simulink library "slib_spectrum_analyser"  (R2020a)
settings: Solver=VariableStepAuto  StartTime=0.0  StopTime=10.0  RelTol=1e-3
libraries: hdlsllib x104, simulink x55, dsphdlxfrm x11, $bdroot x5
(part 3 of 3)

== system slib_spectrum_analyser/SSR Subset Converter/SSR Serializer Imag/Vector to SSR ==
  Vector : Inport
  Bit Concat : hdlsllib/Logic and Bit Operations/Bit Concat  numInputs=8
  Selector0 : Selector  InputPortWidth=8  IndexOptions=Index vector (dialog)  Indices=8  OutputSizes=1
  Selector1 : Selector  InputPortWidth=8  IndexOptions=Index vector (dialog)  Indices=7  OutputSizes=1
  Selector2 : Selector  InputPortWidth=8  IndexOptions=Index vector (dialog)  Indices=6  OutputSizes=1
  Selector3 : Selector  InputPortWidth=8  IndexOptions=Index vector (dialog)  Indices=5  OutputSizes=1
  Selector4 : Selector  InputPortWidth=8  IndexOptions=Index vector (dialog)  Indices=4  OutputSizes=1
  Selector5 : Selector  InputPortWidth=8  IndexOptions=Index vector (dialog)  Indices=3  OutputSizes=1
  Selector6 : Selector  InputPortWidth=8  IndexOptions=Index vector (dialog)  Indices=2  OutputSizes=1
  Selector7 : Selector  InputPortWidth=8  IndexOptions=Index vector (dialog)  Indices=1  OutputSizes=1
  SSR : Outport
  wires:
  Selector7/1 -> Bit Concat/8
  Selector6/1 -> Bit Concat/7
  Selector5/1 -> Bit Concat/6
  Selector4/1 -> Bit Concat/5
  Selector3/1 -> Bit Concat/4
  Selector2/1 -> Bit Concat/3
  Selector1/1 -> Bit Concat/2
  Selector0/1 -> Bit Concat/1
  Vector/1 -> Selector0/1, Selector1/1, Selector2/1, Selector3/1, Selector4/1, Selector5/1, Selector7/1, Selector6/1
  Bit Concat/1 -> SSR/1

== system slib_spectrum_analyser/SSR Subset Converter/SSR Serializer Real/SSR to Vector ==
  SSR : Inport
  Bit Slice0 : hdlsllib/Logic and Bit Operations/Bit Slice  lidx=15  ridx=0
      settings: SourceProductBaseCode=SL
  Bit Slice1 : hdlsllib/Logic and Bit Operations/Bit Slice  lidx=31  ridx=16
      settings: SourceProductBaseCode=SL
  Bit Slice2 : hdlsllib/Logic and Bit Operations/Bit Slice  lidx=47  ridx=32
      settings: SourceProductBaseCode=SL
  Bit Slice3 : hdlsllib/Logic and Bit Operations/Bit Slice  lidx=63  ridx=48
      settings: SourceProductBaseCode=SL
  Bit Slice4 : hdlsllib/Logic and Bit Operations/Bit Slice  lidx=79  ridx=64
      settings: SourceProductBaseCode=SL
  Bit Slice5 : hdlsllib/Logic and Bit Operations/Bit Slice  lidx=95  ridx=80
      settings: SourceProductBaseCode=SL
  Bit Slice6 : hdlsllib/Logic and Bit Operations/Bit Slice  lidx=111  ridx=96
      settings: SourceProductBaseCode=SL
  Bit Slice7 : hdlsllib/Logic and Bit Operations/Bit Slice  lidx=127  ridx=112
      settings: SourceProductBaseCode=SL
  Matrix Concatenate : Concatenate  NumInputs=8  ConcatenateDimension=2
  Vector : Outport
  wires:
  Matrix Concatenate/1 -> Vector/1
  SSR/1 -> Bit Slice6/1, Bit Slice7/1, Bit Slice5/1, Bit Slice4/1, Bit Slice3/1, Bit Slice2/1, Bit Slice1/1, Bit Slice0/1
  Bit Slice0/1 -> Matrix Concatenate/1
  Bit Slice1/1 -> Matrix Concatenate/2
  Bit Slice2/1 -> Matrix Concatenate/3
  Bit Slice3/1 -> Matrix Concatenate/4
  Bit Slice4/1 -> Matrix Concatenate/5
  Bit Slice5/1 -> Matrix Concatenate/6
  Bit Slice6/1 -> Matrix Concatenate/7
  Bit Slice7/1 -> Matrix Concatenate/8

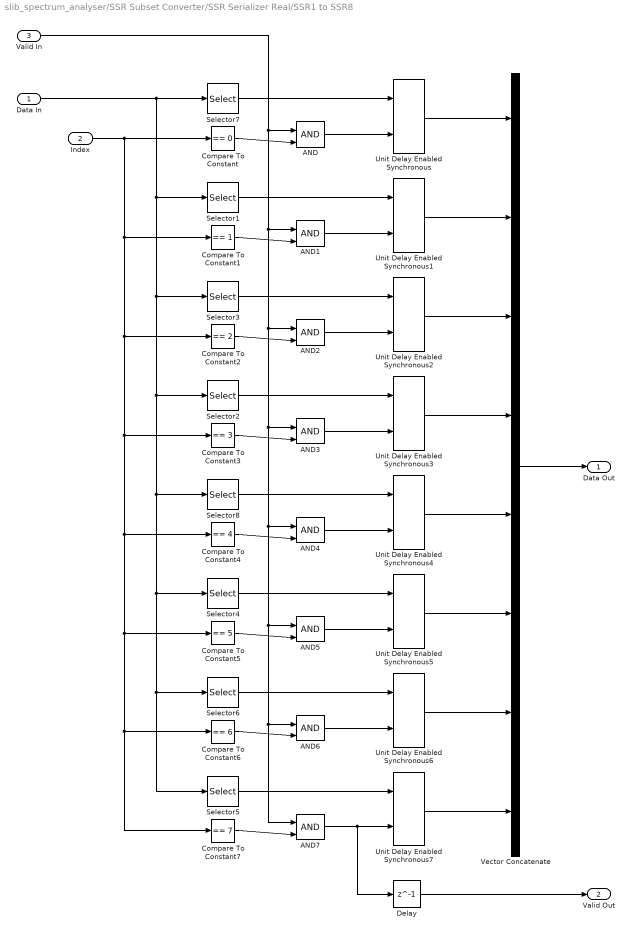
== system slib_spectrum_analyser/SSR Subset Converter/SSR Serializer Real/SSR1 to SSR8 ==
  Data In : Inport
  Index : Inport  Port=2
  Valid In : Inport  Port=3
  AND{,1..7} (8 alike) : Logic  IconShape=distinctive  AllPortsSameDT=off  OutDataTypeStr=boolean
  Compare To Constant : simulink/Logic and Bit Operations/Compare To Constant  relop===  const=0  OutDataTypeStr=boolean
  Compare To Constant1 : simulink/Logic and Bit Operations/Compare To Constant  relop===  const=1  OutDataTypeStr=boolean
  Compare To Constant2 : simulink/Logic and Bit Operations/Compare To Constant  relop===  const=2  OutDataTypeStr=boolean
  Compare To Constant3 : simulink/Logic and Bit Operations/Compare To Constant  relop===  const=3  OutDataTypeStr=boolean
  Compare To Constant4 : simulink/Logic and Bit Operations/Compare To Constant  relop===  const=4  OutDataTypeStr=boolean
  Compare To Constant5 : simulink/Logic and Bit Operations/Compare To Constant  relop===  const=5  OutDataTypeStr=boolean
  Compare To Constant6 : simulink/Logic and Bit Operations/Compare To Constant  relop===  const=6  OutDataTypeStr=boolean
  Compare To Constant7 : simulink/Logic and Bit Operations/Compare To Constant  relop===  const=7  OutDataTypeStr=boolean
  Delay : Delay  DelayLength=1
  Selector{1..8} (8 alike) : Selector  IndexMode=Zero-based  InputPortWidth=8  IndexOptions=Index vector (dialog)  Indices=0  OutputSizes=1
  Unit Delay Enabled Synchronous{,1..7} (8 alike) : hdlsllib/Discrete/Unit Delay Enabled Synchronous  InitialCondition=0.0  SampleTime=-1
      settings: SourceProductBaseCode=SL
  Vector Concatenate : Concatenate  NumInputs=8
  Data Out : Outport
  Valid Out : Outport  Port=2
  wires:
  Compare To Constant1/1 -> AND1/2
  Compare To Constant2/1 -> AND2/2
  Compare To Constant3/1 -> AND3/2
  Compare To Constant4/1 -> AND4/2
  Compare To Constant5/1 -> AND5/2
  Compare To Constant6/1 -> AND6/2
  Compare To Constant7/1 -> AND7/2
  AND7/1 -> Delay/1, Unit Delay Enabled Synchronous7/2
  AND6/1 -> Unit Delay Enabled Synchronous6/2
  AND5/1 -> Unit Delay Enabled Synchronous5/2
  AND4/1 -> Unit Delay Enabled Synchronous4/2
  AND3/1 -> Unit Delay Enabled Synchronous3/2
  AND2/1 -> Unit Delay Enabled Synchronous2/2
  AND1/1 -> Unit Delay Enabled Synchronous1/2
  Valid In/1 -> AND/1, AND1/1, AND2/1, AND3/1, AND4/1, AND5/1, AND6/1, AND7/1
  Compare To Constant/1 -> AND/2
  AND/1 -> Unit Delay Enabled Synchronous/2
  Selector3/1 -> Unit Delay Enabled Synchronous2/1
  Selector6/1 -> Unit Delay Enabled Synchronous6/1
  Data In/1 -> Selector5/1, Selector6/1, Selector4/1, Selector8/1, Selector2/1, Selector3/1, Selector1/1, Selector7/1
  Selector2/1 -> Unit Delay Enabled Synchronous3/1
  Selector7/1 -> Unit Delay Enabled Synchronous/1
  Selector1/1 -> Unit Delay Enabled Synchronous1/1
  Selector5/1 -> Unit Delay Enabled Synchronous7/1
  Index/1 -> Compare To Constant7/1, Compare To Constant6/1, Compare To Constant5/1, Compare To Constant4/1, Compare To Constant3/1, Compare To Constant2/1, Compare To Constant1/1, Compare To Constant/1
  Selector8/1 -> Unit Delay Enabled Synchronous4/1
  Selector4/1 -> Unit Delay Enabled Synchronous5/1
  Vector Concatenate/1 -> Data Out/1
  Delay/1 -> Valid Out/1
  Unit Delay Enabled Synchronous7/1 -> Vector Concatenate/8
  Unit Delay Enabled Synchronous6/1 -> Vector Concatenate/7
  Unit Delay Enabled Synchronous5/1 -> Vector Concatenate/6
  Unit Delay Enabled Synchronous4/1 -> Vector Concatenate/5
  Unit Delay Enabled Synchronous3/1 -> Vector Concatenate/4
  Unit Delay Enabled Synchronous2/1 -> Vector Concatenate/3
  Unit Delay Enabled Synchronous1/1 -> Vector Concatenate/2
  Unit Delay Enabled Synchronous/1 -> Vector Concatenate/1

== system slib_spectrum_analyser/SSR Subset Converter/SSR Serializer Real/SSR2 to SSR8 ==
  Data In : Inport
  Index : Inport  Port=2
  Valid In : Inport  Port=3
  AND{,1..3} (4 alike) : Logic  IconShape=distinctive  AllPortsSameDT=off  OutDataTypeStr=boolean
  Compare To Constant10 : simulink/Logic and Bit Operations/Compare To Constant  relop===  const=2  OutDataTypeStr=boolean
  Compare To Constant11 : simulink/Logic and Bit Operations/Compare To Constant  relop===  const=3  OutDataTypeStr=boolean
  Compare To Constant8 : simulink/Logic and Bit Operations/Compare To Constant  relop===  const=0  OutDataTypeStr=boolean
  Compare To Constant9 : simulink/Logic and Bit Operations/Compare To Constant  relop===  const=1  OutDataTypeStr=boolean
  Delay : Delay  DelayLength=1
  Selector{9..12} (4 alike) : Selector  IndexMode=Zero-based  InputPortWidth=8  IndexOptions=Index vector (dialog)  Indices=[0, 1]  OutputSizes=1
  Unit Delay Enabled Synchronous{,1..3} (4 alike) : hdlsllib/Discrete/Unit Delay Enabled Synchronous  InitialCondition=0.0  SampleTime=-1
      settings: SourceProductBaseCode=SL
  Vector Concatenate : Concatenate  NumInputs=4
  Data Out : Outport
  Valid Out : Outport  Port=2
  wires:
  Compare To Constant11/1 -> AND3/2
  Compare To Constant10/1 -> AND2/2
  Valid In/1 -> AND/1, AND1/1, AND2/1, AND3/1
  Compare To Constant8/1 -> AND/2
  Compare To Constant9/1 -> AND1/2
  AND1/1 -> Unit Delay Enabled Synchronous1/2
  AND2/1 -> Unit Delay Enabled Synchronous2/2
  AND3/1 -> Delay/1, Unit Delay Enabled Synchronous3/2
  AND/1 -> Unit Delay Enabled Synchronous/2
  Selector10/1 -> Unit Delay Enabled Synchronous2/1
  Data In/1 -> Selector9/1, Selector10/1, Selector11/1, Selector12/1
  Selector9/1 -> Unit Delay Enabled Synchronous1/1
  Vector Concatenate/1 -> Data Out/1
  Index/1 -> Compare To Constant11/1, Compare To Constant10/1, Compare To Constant9/1, Compare To Constant8/1
  Selector12/1 -> Unit Delay Enabled Synchronous/1
  Selector11/1 -> Unit Delay Enabled Synchronous3/1
  Delay/1 -> Valid Out/1
  Unit Delay Enabled Synchronous/1 -> Vector Concatenate/1
  Unit Delay Enabled Synchronous1/1 -> Vector Concatenate/2
  Unit Delay Enabled Synchronous2/1 -> Vector Concatenate/3
  Unit Delay Enabled Synchronous3/1 -> Vector Concatenate/4

== system slib_spectrum_analyser/SSR Subset Converter/SSR Serializer Real/SSR4 to SSR8 ==
  Data In : Inport
  Index : Inport  Port=2
  Valid In : Inport  Port=3
  AND : Logic  IconShape=distinctive  AllPortsSameDT=off  OutDataTypeStr=boolean
  AND1 : Logic  IconShape=distinctive  AllPortsSameDT=off  OutDataTypeStr=boolean
  Compare To Constant12 : simulink/Logic and Bit Operations/Compare To Constant  relop===  const=0  OutDataTypeStr=boolean
  Compare To Constant13 : simulink/Logic and Bit Operations/Compare To Constant  relop===  const=1  OutDataTypeStr=boolean
  Delay : Delay  DelayLength=1
  Selector13 : Selector  IndexMode=Zero-based  InputPortWidth=8  IndexOptions=Index vector (dialog)  Indices=[0, 1, 2, 3]  OutputSizes=1
  Selector14 : Selector  IndexMode=Zero-based  InputPortWidth=8  IndexOptions=Index vector (dialog)  Indices=[0, 1, 2, 3]  OutputSizes=1
  Unit Delay Enabled Synchronous : hdlsllib/Discrete/Unit Delay Enabled Synchronous  InitialCondition=0.0  SampleTime=-1
      settings: SourceProductBaseCode=SL
  Unit Delay Enabled Synchronous1 : hdlsllib/Discrete/Unit Delay Enabled Synchronous  InitialCondition=0.0  SampleTime=-1
      settings: SourceProductBaseCode=SL
  Vector Concatenate : Concatenate
  Data Out : Outport
  Valid Out : Outport  Port=2
  wires:
  Compare To Constant13/1 -> AND1/2
  AND1/1 -> Delay/1, Unit Delay Enabled Synchronous1/2
  Valid In/1 -> AND/1, AND1/1
  Compare To Constant12/1 -> AND/2
  AND/1 -> Unit Delay Enabled Synchronous/2
  Index/1 -> Compare To Constant12/1, Compare To Constant13/1
  Selector14/1 -> Unit Delay Enabled Synchronous1/1
  Selector13/1 -> Unit Delay Enabled Synchronous/1
  Data In/1 -> Selector13/1, Selector14/1
  Vector Concatenate/1 -> Data Out/1
  Unit Delay Enabled Synchronous/1 -> Vector Concatenate/1
  Unit Delay Enabled Synchronous1/1 -> Vector Concatenate/2
  Delay/1 -> Valid Out/1

== system slib_spectrum_analyser/SSR Subset Converter/SSR Serializer Real/Vector to SSR ==
  Vector : Inport
  Bit Concat : hdlsllib/Logic and Bit Operations/Bit Concat  numInputs=8
  Selector0 : Selector  InputPortWidth=8  IndexOptions=Index vector (dialog)  Indices=8  OutputSizes=1
  Selector1 : Selector  InputPortWidth=8  IndexOptions=Index vector (dialog)  Indices=7  OutputSizes=1
  Selector2 : Selector  InputPortWidth=8  IndexOptions=Index vector (dialog)  Indices=6  OutputSizes=1
  Selector3 : Selector  InputPortWidth=8  IndexOptions=Index vector (dialog)  Indices=5  OutputSizes=1
  Selector4 : Selector  InputPortWidth=8  IndexOptions=Index vector (dialog)  Indices=4  OutputSizes=1
  Selector5 : Selector  InputPortWidth=8  IndexOptions=Index vector (dialog)  Indices=3  OutputSizes=1
  Selector6 : Selector  InputPortWidth=8  IndexOptions=Index vector (dialog)  Indices=2  OutputSizes=1
  Selector7 : Selector  InputPortWidth=8  IndexOptions=Index vector (dialog)  Indices=1  OutputSizes=1
  SSR : Outport
  wires:
  Bit Concat/1 -> SSR/1
  Vector/1 -> Selector6/1, Selector7/1, Selector5/1, Selector4/1, Selector3/1, Selector2/1, Selector1/1, Selector0/1
  Selector0/1 -> Bit Concat/1
  Selector1/1 -> Bit Concat/2
  Selector2/1 -> Bit Concat/3
  Selector3/1 -> Bit Concat/4
  Selector4/1 -> Bit Concat/5
  Selector5/1 -> Bit Concat/6
  Selector6/1 -> Bit Concat/7
  Selector7/1 -> Bit Concat/8

== matlab function slib_spectrum_analyser/Direct Memory Access/Direct Memory Access/DDR Communication/Write Controller ==
  data: valid input; count input; push output boolean; pop output; length input; enable input; start input boolean; wr_complete input; wr_ready input; wr_len output; buffer output; state output; empty input; debug_count output
function [push, pop, wr_len, buffer, state, debug_count] = ddr_write_control(valid, count, length, enable, start, wr_complete, wr_ready, empty)

% Create persistent variables (registers)
persistent burst_count;
persistent time_count;
persistent current_state;
persistent buffer_pointer;

if(isempty(burst_count))
    burst_count = fi(0, 0, 16, 0);
end

if(isempty(time_count))
    time_count = fi(0, 0, 32, 0);
end

if(isempty(current_state))
    current_state = fi(0, 0, 4, 0);
end

if(isempty(buffer_pointer))
    buffer_pointer = fi(0, 0, 2, 0);
end

% FSM States
IDLE  = fi(0, 0, 4, 0);
START = fi(1, 0, 4, 0);
COUNT = fi(2, 0, 4, 0);
WAIT  = fi(4, 0, 4, 0);

switch current_state
    case IDLE
        push = false;
        pop = wr_ready;
        wr_len = length;
        buffer = buffer_pointer;
        state = current_state;
        debug_count = burst_count;
        
        burst_count = fi(0, 0, 16, 0);
        
        if enable && time_count >= count
            current_state = START;
            time_count = fi(0, 0, 32, 0);
        else
            current_state = IDLE;
            if time_count < count
                time_count = fi(time_count + 1, 0, 32, 0);
            end
        end
        
    case START
        pop = false;
        wr_len = length;
        buffer = buffer_pointer;
        state = current_state;
        debug_count = burst_count;
        
        if ~enable
            push = false;
            burst_count = fi(0, 0, 16, 0);
            current_state = IDLE;
        else
            if start && valid
                push = true;
                burst_count = fi(burst_count + 1, 0, 16, 0);
                current_state = COUNT;
            else
                push = false;
                burst_count = fi(0, 0, 16, 0);
                current_state = START;
            end
        end            
        
    case COUNT
        pop = false;
        wr_len = length;
        buffer = buffer_pointer;
        state = current_state;
        debug_count = burst_count;
        
        if valid
            push = true;
            burst_count = fi(burst_count + 1, 0, 16, 0);
        else
            push = false;
        end
        
        if burst_count >= length
            current_state = WAIT;
            if buffer_pointer > fi(1, 0, 2, 0)
                buffer_pointer = fi(0, 0, 2, 0);
            else
            	buffer_pointer = fi(buffer_pointer+1, 0, 2, 0);
            end
        else
            current_state = COUNT;
        end
        
    case WAIT
        push = false;
        pop = wr_ready;
        wr_len = length;
        buffer = buffer_pointer;
        state = current_state;
        debug_count = burst_count;
        
        burst_count = fi(0, 0, 16, 0);
        
        if empty && wr_complete
            current_state = IDLE;
        else
            current_state = WAIT;
        end
        
    otherwise
        push = false;
        pop = wr_ready;
        wr_len = length;
        buffer = buffer_pointer;
        state = current_state;
        debug_count = burst_count;
        
        burst_count = fi(0, 0, 16, 0);
        
        current_state = IDLE;
        
end

== matlab function slib_spectrum_analyser/Preprocessing Window/Direct Memory Access/DDR Read Controller ==
  data: valid_out output boolean; count_out output; ready_out output boolean; length_in input; address input; start input boolean; rd_aready input; rd_dvalid input; rd_addr output uint32; rd_len output; rd_avalid output
function [valid_out,count_out,ready_out,rd_addr,rd_len,rd_avalid] = ddr_read_control(length_in, address, start, rd_aready, rd_dvalid)

% Create persistent variables (registers)
persistent burst_stop
if(isempty(burst_stop))
    burst_stop = uint16(0);
end
persistent burst_count;
if(isempty(burst_count))
    burst_count = uint16(0);
end
persistent rstate;
if isempty(rstate)
    rstate = fi(0, 0, 4, 0);
end


% State Memory Encoding
IDLE             = fi(1, 0, 4, 0);
READ_BURST_START = fi(2, 0, 4, 0);
DATA_COUNT       = fi(4, 0, 4, 0);

% Read control state machine
switch (rstate)
    case IDLE
        % output to AXI4 Master
        rd_addr = address;
        rd_len = uint16(0);
        rd_avalid = false;
        
        % output to DUT
        valid_out = false;
        ready_out = true;
        count_out = uint16(0);
        
        % State vars
        burst_count = uint16(0);
        burst_stop = uint16(length_in);
        
        if rd_aready && start
            rstate(:) = READ_BURST_START;
        end
        
    case READ_BURST_START
        % output to AXI4 Master
        rd_addr = address;
        rd_len = uint16(burst_stop);
        rd_avalid = true;
        
        % output to DUT
        valid_out = false;
        count_out = uint16(0);
        ready_out = false;
        
        rstate(:) = DATA_COUNT;
        
    case DATA_COUNT
        % output to AXI4 Master
        rd_addr = address;
        rd_len = uint16(burst_stop);
        rd_avalid = false;
        
        % output to DUT
        valid_out = rd_dvalid;
        count_out = uint16(burst_count);
        ready_out = false;
        
        % State vars
        if ( rd_dvalid )
            burst_count = uint16(burst_count + 1);
        end
        
        if ( burst_count == burst_stop )
            rstate(:) = IDLE;
        else
            rstate(:) = DATA_COUNT;
        end
        
    otherwise
        % output to AXI4 Master
        rd_addr = uint32(0);
        rd_len = uint16(0);
        rd_avalid = false;
        
        % output to DUT
        valid_out = false;
        count_out = uint16(0);
        ready_out = false;
        
        rstate(:) = IDLE;
end

end
